simulink model "System"  (R2015b)
settings: Solver=FixedStepAuto  StartTime=0.0  StopTime=10.0  FixedStep=0.1  RelTol=1e-3
settings Model: Creator=Deepak  LastModifiedBy=Deepak
settings ModelReferenceCC: ModelReferenceMinAlgLoopOccurrences=on

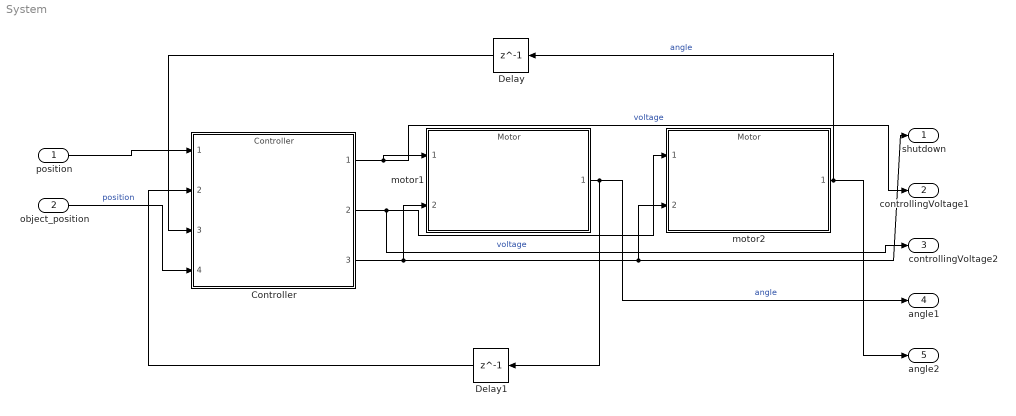
== system System ==
  position : Inport
  object_position : Inport  Port=2
      settings: AttributesFormatString=position
  Controller : ModelReference  ModelNameDialog=Controller  SimulationMode=Normal  ModelReferenceVersion=1.38  CopyOfModelName=Controller
  Delay : Delay  DelayLength=1  InitialCondition=0
  Delay1 : Delay  DelayLength=1  InitialCondition=0
  motor1 : ModelReference  ModelNameDialog=Motor  SimulationMode=Normal  ModelReferenceVersion=1.7  CopyOfModelName=Motor
  motor2 : ModelReference  ModelNameDialog=Motor  SimulationMode=Normal  ModelReferenceVersion=1.7  CopyOfModelName=Motor
  shutdown : Outport
  controllingVoltage1 : Outport  Port=2
      settings: AttributesFormatString=voltage
  controllingVoltage2 : Outport  Port=3
      settings: AttributesFormatString=voltage
  angle1 : Outport  Port=4
      settings: AttributesFormatString=angle
  angle2 : Outport  Port=5
      settings: AttributesFormatString=angle
  wires:
  Controller/1 -> motor1/1, controllingVoltage1/1  "voltage"
  Controller/2 -> motor2/1, controllingVoltage2/1  "voltage"
  Controller/3 -> shutdown/1, motor2/2, motor1/2
  motor1/1 -> Delay1/1, angle1/1  "angle"
  motor2/1 -> Delay/1, angle2/1  "angle"
  object_position/1 -> Controller/4  "position"
  position/1 -> Controller/1
  Delay/1 -> Controller/3
  Delay1/1 -> Controller/2
